simulink model "Lab4_model"  (R2017b)
settings: Solver=VariableStepAuto  StartTime=0.0  StopTime=5000  RelTol=1e-3
values from neighbouring files (symbols this model uses):
  Ts = Ts1/10    (= 30)    [Lab_4.m]
undefined symbols (not defined in the file or in its folder): den_final, den_final_cor, num_final, num_final_cor
libraries: cstblocks x6
settings Model: Creator=kelem  LastModifiedBy=kelem

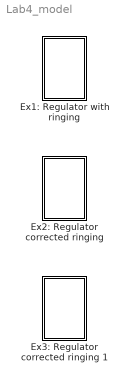
== system Lab4_model ==
  Ex1: Regulator with ringing : Subsystem
  "Ex2: Regulator corrected ringing " : Subsystem
  Ex3: Regulator corrected ringing 1 : Subsystem

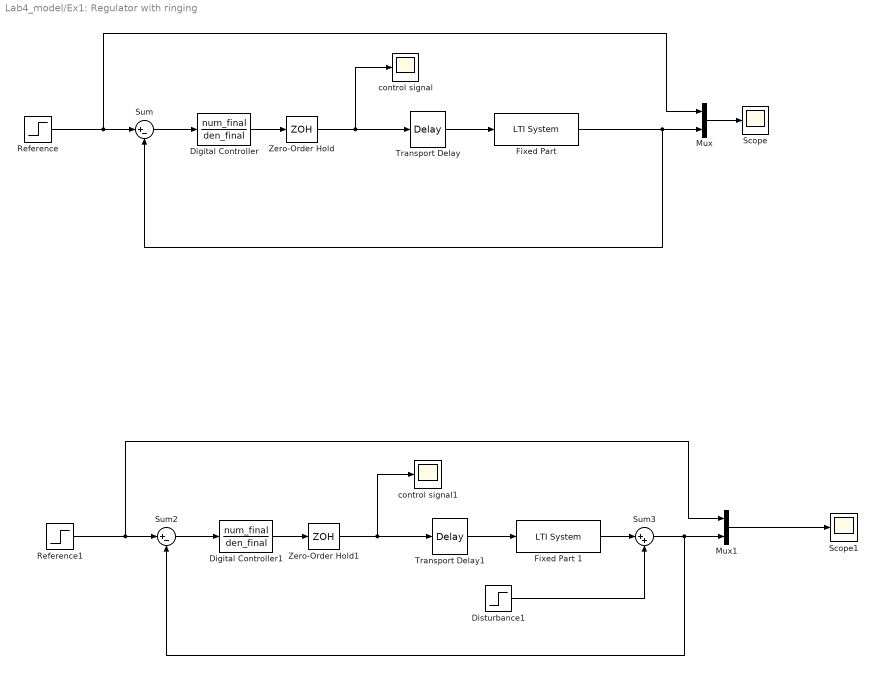
== system Lab4_model/Ex1: Regulator with ringing ==
  Digital Controller : DiscreteTransferFcn  Numerator=num_final  Denominator=den_final  SampleTime=Ts
  Digital Controller1 : DiscreteTransferFcn  Numerator=num_final  Denominator=den_final  SampleTime=Ts
  Disturbance1 : Step  SampleTime=50
  "Fixed Part " : cstblocks/LTI System  sys=Hf  IC=[]
  Fixed Part 1 : cstblocks/LTI System  sys=Hf  IC=[]
  Mux : Mux  Inputs=2
  Mux1 : Mux  Inputs=2
  Reference : Step  SampleTime=0
  Reference1 : Step  SampleTime=0
  Scope : Scope
  Scope1 : Scope
  Sum : Sum  Inputs=|+-
  Sum2 : Sum  Inputs=|+-
  Sum3 : Sum  Inputs=|++
  Transport Delay : TransportDelay
  Transport Delay1 : TransportDelay
  Zero-Order Hold : ZeroOrderHold  SampleTime=-1
  Zero-Order Hold1 : ZeroOrderHold  SampleTime=-1
  control signal : Scope
  control signal1 : Scope
  wires:
  Sum/1 -> Digital Controller/1
  "Fixed Part "/1 -> Sum/2, Mux/2
  Mux/1 -> Scope/1
  Sum3/1 -> Sum2/2, Mux1/2
  Digital Controller1/1 -> Zero-Order Hold1/1
  Sum2/1 -> Digital Controller1/1
  Fixed Part 1/1 -> Sum3/1
  Disturbance1/1 -> Sum3/2
  Reference1/1 -> Mux1/1, Sum2/1
  Transport Delay1/1 -> Fixed Part 1/1
  Mux1/1 -> Scope1/1
  Zero-Order Hold1/1 -> control signal1/1, Transport Delay1/1
  Zero-Order Hold/1 -> control signal/1, Transport Delay/1
  Transport Delay/1 -> "Fixed Part "/1
  Reference/1 -> Mux/1, Sum/1
  Digital Controller/1 -> Zero-Order Hold/1

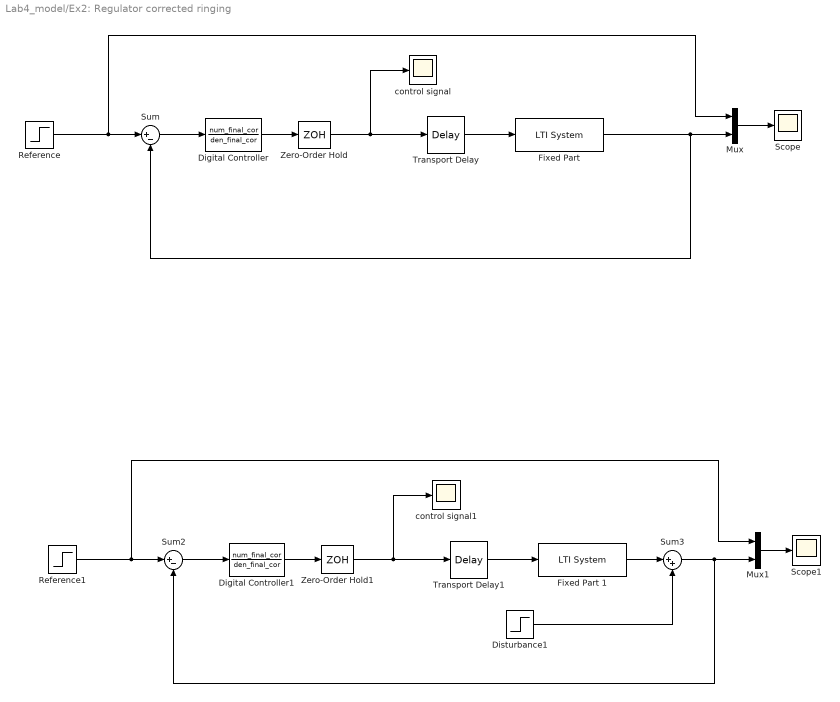
== system Lab4_model/Ex2: Regulator corrected ringing  ==
  Digital Controller : DiscreteTransferFcn  Numerator=num_final_cor  Denominator=den_final_cor  SampleTime=Ts
  Digital Controller1 : DiscreteTransferFcn  Numerator=num_final_cor  Denominator=den_final_cor  SampleTime=Ts
  Disturbance1 : Step  SampleTime=50
  "Fixed Part " : cstblocks/LTI System  sys=Hf  IC=[]
  Fixed Part 1 : cstblocks/LTI System  sys=Hf  IC=[]
  Mux : Mux  Inputs=2
  Mux1 : Mux  Inputs=2
  Reference : Step  SampleTime=0
  Reference1 : Step  SampleTime=0
  Scope : Scope
  Scope1 : Scope
  Sum : Sum  Inputs=|+-
  Sum2 : Sum  Inputs=|+-
  Sum3 : Sum  Inputs=|++
  Transport Delay : TransportDelay
  Transport Delay1 : TransportDelay
  Zero-Order Hold : ZeroOrderHold  SampleTime=-1
  Zero-Order Hold1 : ZeroOrderHold  SampleTime=-1
  control signal : Scope
  control signal1 : Scope
  wires:
  Sum/1 -> Digital Controller/1
  "Fixed Part "/1 -> Sum/2, Mux/2
  Mux/1 -> Scope/1
  Digital Controller1/1 -> Zero-Order Hold1/1
  Sum2/1 -> Digital Controller1/1
  Fixed Part 1/1 -> Sum3/1
  Disturbance1/1 -> Sum3/2
  Reference1/1 -> Mux1/1, Sum2/1
  Transport Delay1/1 -> Fixed Part 1/1
  Mux1/1 -> Scope1/1
  Zero-Order Hold1/1 -> control signal1/1, Transport Delay1/1
  Zero-Order Hold/1 -> control signal/1, Transport Delay/1
  Transport Delay/1 -> "Fixed Part "/1
  Reference/1 -> Mux/1, Sum/1
  Digital Controller/1 -> Zero-Order Hold/1
  Sum3/1 -> Sum2/2, Mux1/2

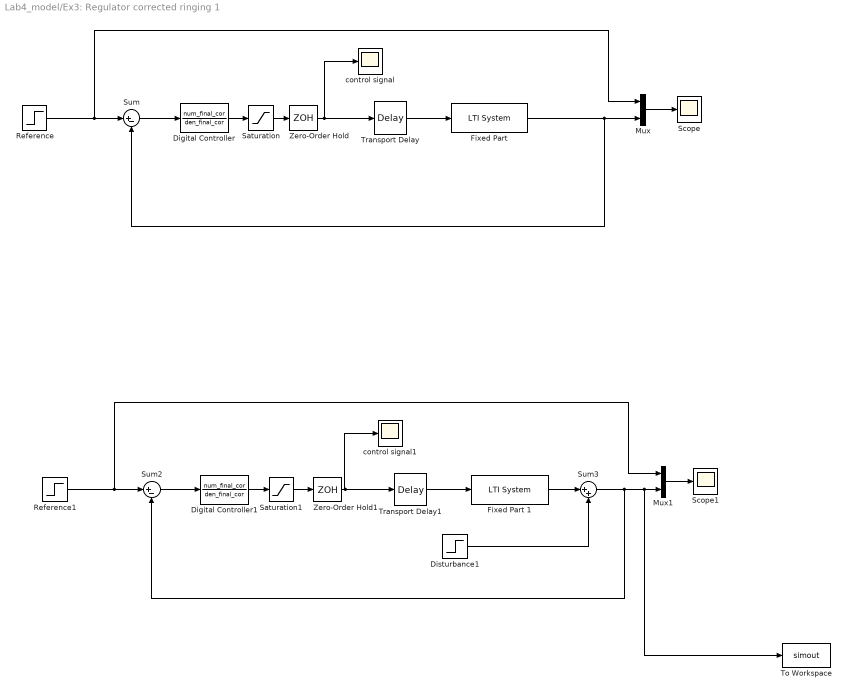
== system Lab4_model/Ex3: Regulator corrected ringing 1 ==
  Digital Controller : DiscreteTransferFcn  Numerator=num_final_cor  Denominator=den_final_cor  SampleTime=Ts
  Digital Controller1 : DiscreteTransferFcn  Numerator=num_final_cor  Denominator=den_final_cor  SampleTime=Ts
  Disturbance1 : Step  SampleTime=50
  "Fixed Part " : cstblocks/LTI System  sys=Hf  IC=[]
  Fixed Part 1 : cstblocks/LTI System  sys=Hf  IC=[]
  Mux : Mux  Inputs=2
  Mux1 : Mux  Inputs=2
  Reference : Step  SampleTime=0
  Reference1 : Step  SampleTime=0
  Saturation : Saturate  UpperLimit=0.6  LowerLimit=0
  Saturation1 : Saturate  UpperLimit=0.6  LowerLimit=0
  Scope : Scope
  Scope1 : Scope
  Sum : Sum  Inputs=|+-
  Sum2 : Sum  Inputs=|+-
  Sum3 : Sum  Inputs=|++
  To Workspace : ToWorkspace  VariableName=simout  SaveFormat=Timeseries  SampleTime=-1
  Transport Delay : TransportDelay
  Transport Delay1 : TransportDelay
  Zero-Order Hold : ZeroOrderHold  SampleTime=-1
  Zero-Order Hold1 : ZeroOrderHold  SampleTime=-1
  control signal : Scope
  control signal1 : Scope
  wires:
  Sum/1 -> Digital Controller/1
  "Fixed Part "/1 -> Sum/2, Mux/2
  Mux/1 -> Scope/1
  Digital Controller1/1 -> Saturation1/1
  Sum2/1 -> Digital Controller1/1
  Fixed Part 1/1 -> Sum3/1
  Disturbance1/1 -> Sum3/2
  Reference1/1 -> Mux1/1, Sum2/1
  Transport Delay1/1 -> Fixed Part 1/1
  Mux1/1 -> Scope1/1
  Zero-Order Hold1/1 -> control signal1/1, Transport Delay1/1
  Zero-Order Hold/1 -> control signal/1, Transport Delay/1
  Transport Delay/1 -> "Fixed Part "/1
  Reference/1 -> Mux/1, Sum/1
  Digital Controller/1 -> Saturation/1
  Saturation/1 -> Zero-Order Hold/1
  Saturation1/1 -> Zero-Order Hold1/1
  Sum3/1 -> Sum2/2, To Workspace/1, Mux1/2
